simulink model "testVelocities"  (Simulink 8.7)
settings: Solver=FixedStepDiscrete  StartTime=0.0  StopTime=10  FixedStep=0.01  RelTol=1e-3
InitFcn:
  | WBT_wbiList = 'ROBOT_TORQUE_CONTROL_TEST';
libraries: WBToolboxLibrary x5
settings Model: Creator=DanielePucci  LastModifiedBy=gnava
settings DataIOCC: SaveFormat=Dataset
settings DebuggingCC: UnderspecifiedInitializationDetection=Simplified  MergeDetectMultiDrivingBlocksExec=error  AllowSymbolicDim=off
settings HardwareCC: ProdBitPerPointer=64  ProdLargestAtomicFloat=Float  ProdIntDivRoundTo=Zero  ProdEndianess=LittleEndian  ProdWordSize=64  ProdHWDeviceType=Intel->x86-64 (Windows64)
settings GRTTargetCC: GeneratePreprocessorConditionals=Use local settings
settings ConfigComp: CovModelRefEnable=off

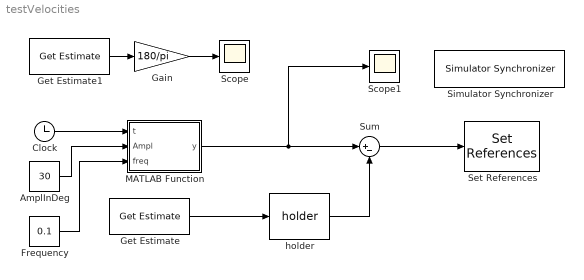
== system testVelocities ==
  AmplInDeg : Constant  Value=30
  Clock : Clock
  Frequency : Constant  Value=0.1
  Gain : Gain  Gain=180/pi
  Get Estimate : WBToolboxLibrary/wholeBodyStates/Get Estimate  estimateType=Joints Position  robotName=WBT_robotName  localName=WBT_modelName  wbiFile=WBT_wbiFilename  wbiList=WBT_wbiList
  Get Estimate1 : WBToolboxLibrary/wholeBodyStates/Get Estimate  estimateType=Joints Velocity  robotName=WBT_robotName  localName=WBT_modelName  wbiFile=WBT_wbiFilename  wbiList=WBT_wbiList
  MATLAB Function : MATLAB Function  TreatAsAtomicUnit=on
  Scope : Scope
  Scope1 : Scope
  Set References : WBToolboxLibrary/wholeBodyActuators/Set References  controlType=Position  robotName=WBT_robotName  localName=WBT_modelName  wbiFile=WBT_wbiFilename  wbiList=WBT_wbiList
  Simulator Synchronizer : WBToolboxLibrary/Utilities/Simulator Synchronizer  period=0.01  serverPortName='/clock/rpc'  clientPortName='/WBT_synchronizer/rpc:o'
  Sum : Sum  Inputs=|+-
  "holder " : WBToolboxLibrary/Utilities/holder 
  wires:
  "holder "/1 -> Sum/2
  Get Estimate/1 -> "holder "/1
  Sum/1 -> Set References/1
  Clock/1 -> MATLAB Function/1(t)
  MATLAB Function/1(y) -> Scope1/1, Sum/1
  Get Estimate1/1 -> Gain/1
  AmplInDeg/1 -> MATLAB Function/2(Ampl)
  Frequency/1 -> MATLAB Function/3(freq)
  Gain/1 -> Scope/1

== matlab function MATLAB Function ==
  data: t input double; y output double; Ampl input double; freq input double
function y = fcn(t,Ampl,freq)
%#codegen

y = Ampl*(pi/180)*sin(2*pi*freq*t);
